simulink model "solarpanel"  (R2023a)
settings: Solver=VariableStepAuto  StartTime=0.0  StopTime=24*3600  RelTol=1e-3
InitFcn:
  | load("sunPositionData.mat")
  | 
  | % Solar Panel
  | m = 50;               % Mass, [kg]
  | w = 1.04;             % Width, [m]
  | l = 1.4;              % Length, [m]
  | d = 0.1;              % Depth, [m]
  | A = w*l;              % Area, [m^2]
  | beta = pi/4;          % Elevation angle, [rad]
  | Kd = 5;               % Damping constant, [N*m/(rad/s)]
  | J = m/12*(l^2*cos(beta)^2+d^2*sin(beta)^2+w^2);  % Inertia, [kg*m^2]
  | 
  | % Motor
  | Kf = 0.07;             % Back EMF cosntant, [V/(rad/s)]
  | Kt = 0.07;             % Torque constant, [N*m/A]
  | L = 1e-5;              % Inductance, [H]
  | R = 8;                % Resistance, [Ohm]
  | Kg = 2000;             % Gear ratio, []
libraries: slpidlib x1
settings Model: PacingRate=501  Creator=drdev  LastModifiedBy=alexa
settings DataIOCC: ExternalInput=[sunTime sunPosition]  LoadExternalInput=on

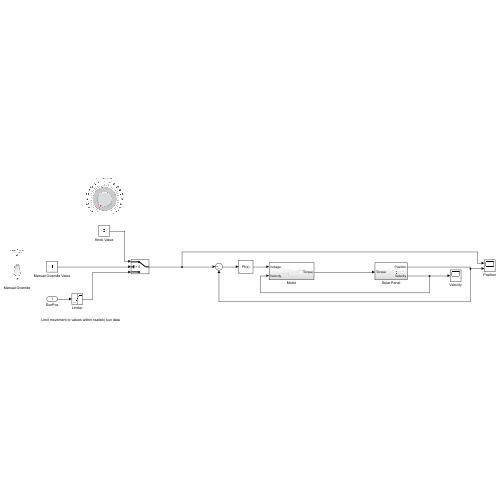
[thumbnail: Simulink's stored preview of the top-level diagram]
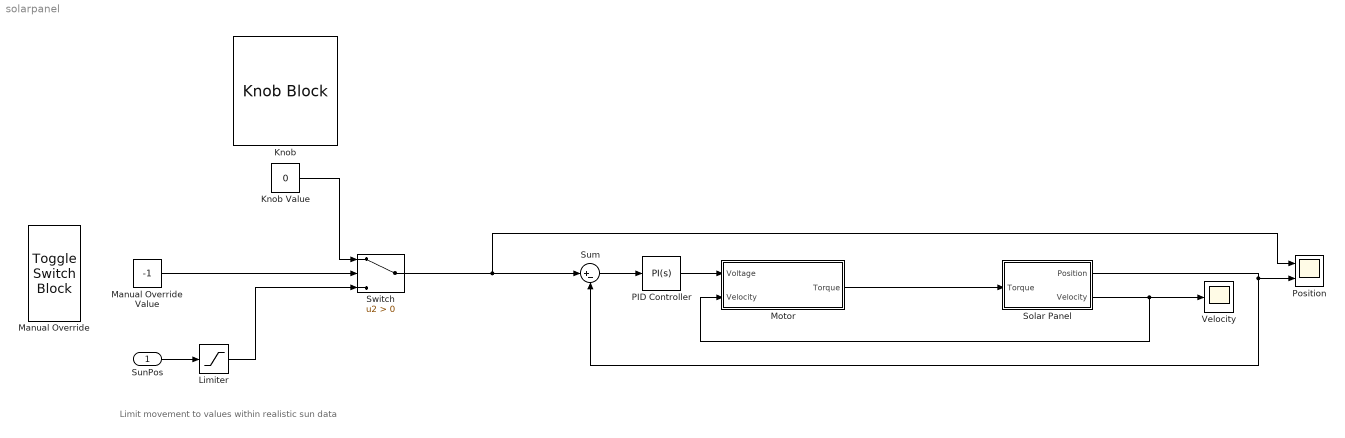
== system solarpanel ==
  note: Limit movement to values within realistic sun data
  SunPos : Inport  Interpolate=off
  Knob : KnobBlock  ScaleMax=6
  Knob Value : Constant  Value=0
  Limiter : Saturate  UpperLimit=6  LowerLimit=1
  Manual Override : ToggleSwitchBlock
      settings: Values={{'Off', 'On'}, [-1 1]}
  Manual Override Value : Constant  Value=-1
  Motor : Subsystem
  PID Controller : slpidlib/PID Controller  Controller=PI  Form=Parallel  TimeDomain=Continuous-time  UseExternalTs=off  SampleTime=-1  IntegratorMethod=Forward Euler  FilterMethod=Forward Euler  ControllerParametersSource=internal  P=400  I=300  UseKiTs=off  D=0  N=100  UseFilter=on  TunerSelectOption=Transfer Function Based (PID Tuner App)  InitialConditionSource=internal  InitialConditionForIntegrator=0  InitialConditionForFilter=0  DifferentiatorICPrevScaledInput=0  ExternalReset=none  TrackingMode=off  Kt=1  LimitOutput=off  SatLimitsSource=internal  UpperSaturationLimit=inf  LowerSaturationLimit=-inf  LinearizeAsGain=on  AntiWindupMode=none  Kb=1  LimitIntegrator=off  UpperIntegratorSaturationLimit=inf  LowerIntegratorSaturationLimit=-inf  POutMin=[]  POutMax=[]  IOutMin=[]  IOutMax=[]  DOutMin=[]  DOutMax=[]  NOutMin=[]  NOutMax=[]  SumOutMin=[]  SumOutMax=[]  SaturationOutMin=[]  SaturationOutMax=[]  PParamMin=[]  PParamMax=[]  IParamMin=[]  IParamMax=[]  DParamMin=[]  DParamMax=[]  NParamMin=[]  NParamMax=[]  KbParamMin=[]  KbParamMax=[]  KtParamMin=[]  KtParamMax=[]  KbOutMin=[]  KbOutMax=[]  KtOutMin=[]  KtOutMax=[]  IntegratorOutMin=[]  IntegratorOutMax=[]  FilterOutMin=[]  FilterOutMax=[]  SumI1OutMin=[]  SumI1OutMax=[]  SumI2OutMin=[]  SumI2OutMax=[]  SumI3OutMin=[]  SumI3OutMax=[]  SumI4OutMin=[]  SumI4OutMax=[]  SumDOutMin=[]  SumDOutMax=[]  DifferentiatorOutMin=[]  DifferentiatorOutMax=[]  FilterDiffOutCoefMin=[]  FilterDiffOutCoefMax=[]  ReciprocalOutMin=[]  ReciprocalOutMax=[]  SumDenOutMin=[]  SumDenOutMax=[]  SumNumOutMin=[]  SumNumOutMax=[]  DivideOutMin=[]  DivideOutMax=[]  UdiffTsProdOutMin=[]  UdiffTsProdOutMax=[]  NTsProdOutMin=[]  NTsProdOutMax=[]  UintegralTsProdOutMin=[]  UintegralTsProdOutMax=[]  UngainTsProdOutMin=[]  UngainTsProdOutMax=[]  ClampingZeroOutDataTypeStr=Inherit: Inherit via back propagation  ClampingZeroOutMin=[]  ClampingZeroOutMax=[]  FilterDenConstantOutDataTypeStr=Inherit: Inherit via back propagation  FilterDenConstantOutMin=[]  FilterDenConstantOutMax=[]  PCopyOutDataTypeStr=Inherit: Inherit via back propagation  PCopyOutMin=[]  PCopyOutMax=[]  NCopyOutDataTypeStr=Inherit: Inherit via back propagation  NCopyOutMin=[]  NCopyOutMax=[]  IntegratorContinuousStateAttributes=''  IntegratorStateMustResolveToSignalObject=off  IntegratorRTWStateStorageClass=Auto  FilterContinuousStateAttributes=''  FilterStateMustResolveToSignalObject=off  FilterRTWStateStorageClass=Auto  ParallelPVariant=InternalParameters  IdealPVariant=Disabled  IVariant=InternalParameters  DVariant=Disabled  IntegratorVariant=Continuous  SatVariant=Disabled  AWVariant=Passthrough  PCopyVariant=Disabled  TRVariant=Disabled  FdbkBlocksVariant=Forward  IdealPFdbkVariant=Disabled  SatFdbkVariant=Disabled  DerivativeFilterVariant=Disabled  NVariant=Disabled  NCopyVariant=Disabled_SignalSpec  FilterICVariant=Disabled  IntegratorICVariant=InternalICs  ExternalResetVariant=Disabled  TRSumVariant=Passthrough  SumFdbkVariant=Disabled  SumVariant=Sum_PI  TsampFilterVariant=InternalTs  TsampNgainVariant=Passthrough  TsampIntegralVariant=Disabled_SignalSpec  ExternalSaturationOutDataTypeStr=Inherit: Same as second input
  Position : Scope  NumInputPorts=2
  Solar Panel : Subsystem
  Sum : Sum  Inputs=|+-
  Switch : Switch  Criteria=u2 > Threshold  SaturateOnIntegerOverflow=off  InputSameDT=off
  Velocity : Scope
  wires:
  Solar Panel/1(Position) -> Sum/2, Position/2
  Solar Panel/2(Velocity) -> Motor/2(Velocity), Velocity/1
  Motor/1(Torque) -> Solar Panel/1(Torque)
  Sum/1 -> PID Controller/1
  PID Controller/1 -> Motor/1(Voltage)
  SunPos/1 -> Limiter/1
  Switch/1 -> Sum/1, Position/1
  Knob Value/1 -> Switch/1
  Manual Override Value/1 -> Switch/2
  Limiter/1 -> Switch/3

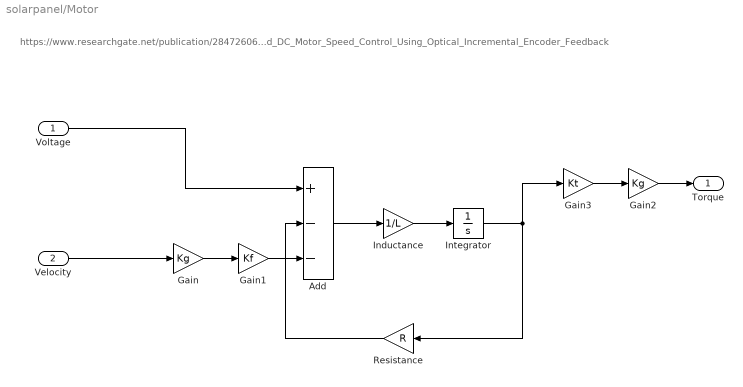
== system solarpanel/Motor ==
  note: https://www.researchgate.net/publication/284726065_Modeling_Simulation_and_Implementation_of_Brushed_DC_Motor_Speed_Control_Using_Optical_Incremental_Encoder_Feedback
  Voltage : Inport
  Velocity : Inport  Port=2
  Add : Sum  Inputs=+--
  Gain : Gain  Gain=Kg
  Gain1 : Gain  Gain=Kf
  Gain2 : Gain  Gain=Kg
  Gain3 : Gain  Gain=Kt
  Inductance : Gain  Gain=1/L
  Integrator : Integrator
  Resistance : Gain  Gain=R
  Torque : Outport
  wires:
  Inductance/1 -> Integrator/1
  Add/1 -> Inductance/1
  Gain/1 -> Gain1/1
  Gain1/1 -> Add/3
  Voltage/1 -> Add/1
  Resistance/1 -> Add/2
  Integrator/1 -> Gain3/1, Resistance/1
  Velocity/1 -> Gain/1
  Gain2/1 -> Torque/1
  Gain3/1 -> Gain2/1

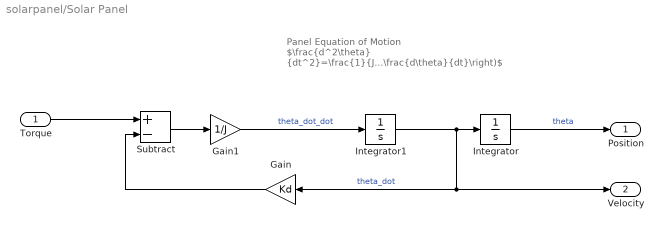
== system solarpanel/Solar Panel ==
  note: Panel Equation of Motion
      | $\frac{d^2\theta} {dt^2}=\frac{1}{J}\left(T-K_d\frac{d\theta}{dt}\right)$
  Torque : Inport
  Gain : Gain  Gain=Kd
  Gain1 : Gain  Gain=1/J
  Integrator : Integrator
  Integrator1 : Integrator
  Subtract : Sum  Inputs=+-
  Position : Outport
  Velocity : Outport  Port=2
  wires:
  Gain1/1 -> Integrator1/1  "theta_dot_dot"
  Subtract/1 -> Gain1/1
  Integrator/1 -> Position/1  "theta"
  Integrator1/1 -> Velocity/1, Gain/1, Integrator/1  "theta_dot"
  Gain/1 -> Subtract/2
  Torque/1 -> Subtract/1
